simulink model "SolarPanelTest"  (R2019a)
settings: Solver=VariableStepAuto  StartTime=0.0  StopTime=10.0  RelTol=1e-3
undefined symbols (not defined in the file): J, Kd
settings Model: Creator=Safet  LastModifiedBy=Safet

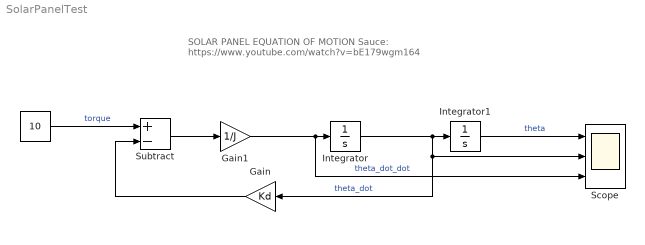
== system SolarPanelTest ==
  note: SOLAR PANEL EQUATION OF MOTION
      |
      | Sauce: https://www.youtube.com/watch?v=bE179wgm164
  " " : Constant  Value=10
  Gain : Gain  Gain=Kd
  Gain1 : Gain  Gain=1/J
  Integrator : Integrator
  Integrator1 : Integrator
  Scope : Scope  NumInputPorts=3
  Subtract : Sum  Inputs=+-
  wires:
  Integrator/1 -> Gain/1, Scope/2, Integrator1/1  "theta_dot"
  Integrator1/1 -> Scope/1  "theta"
  Gain1/1 -> Scope/3, Integrator/1  "theta_dot_dot"
  " "/1 -> Subtract/1  "torque"
  Gain/1 -> Subtract/2
  Subtract/1 -> Gain1/1
